simulink model "main_simulation"  (R2019b)
settings: Solver=VariableStepAuto  StartTime=0.0  StopTime=10.0  RelTol=1e-3
libraries: simulink x1
settings Model: Creator=LBRY-SVC-Patron  LastModifiedBy=logan
settings DataIOCC: ReturnWorkspaceOutputs=off
settings OptimizationCC: UseDivisionForNetSlopeComputation=on
settings DebuggingCC: ArithmeticOperatorsInVariantConditions=warning
settings SFSimCC: SimUseLocalCustomCode=off  CustomCodeUndefinedFunction=UseInterfaceOnly
settings RTWCC: RTWUseLocalCustomCode=off

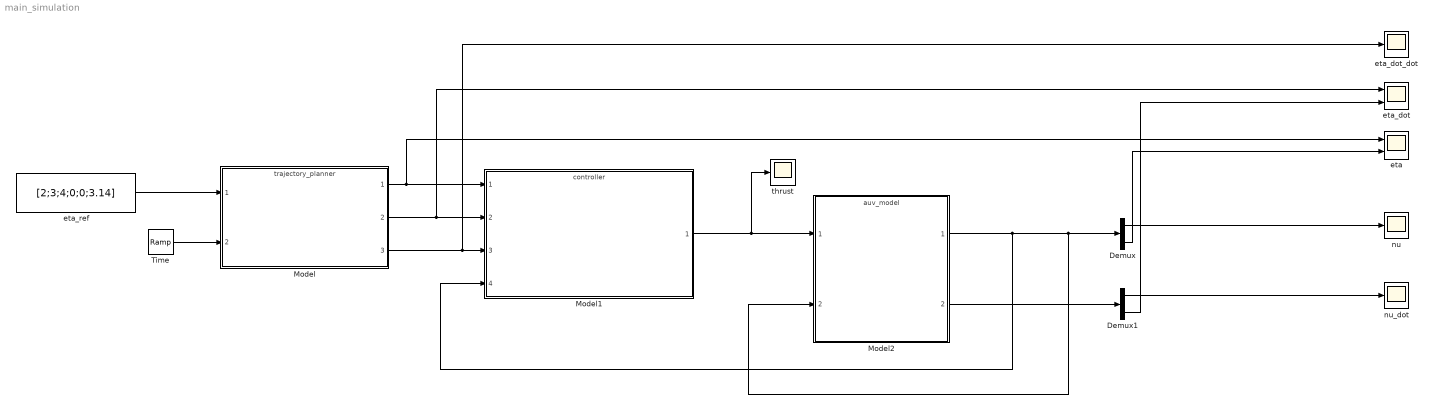
== system main_simulation ==
  Demux : Demux  Outputs=[6,6]
  Demux1 : Demux  Outputs=[6,6]
  Model : ModelReference  ModelNameDialog=trajectory_planner.slx  SimulationMode=Normal  ModelReferenceVersion=1.54
  Model1 : ModelReference  ModelNameDialog=controller.slx  SimulationMode=Normal  ModelReferenceVersion=1.79
  Model2 : ModelReference  ModelNameDialog=auv_model.slx  SimulationMode=Normal  ModelReferenceVersion=1.16
  "Time " : simulink/Sources/Ramp  slope=1  start=0  InitialOutput=0
  eta : Scope  NumInputPorts=2
  eta_dot : Scope  NumInputPorts=2
  eta_dot_dot : Scope
  eta_ref : Constant  Value=[2;3;4;0;0;3.14]
  nu : Scope
  nu_dot : Scope
  "thrust " : Scope
  wires:
  Model/1 -> Model1/1, eta/1
  Model/2 -> Model1/2, eta_dot/1
  "Time "/1 -> Model/2
  eta_ref/1 -> Model/1
  Model2/1 -> Model1/4, Demux/1, Model2/2
  Model1/1 -> "thrust "/1, Model2/1
  Model/3 -> Model1/3, eta_dot_dot/1
  Demux/1 -> nu/1
  Demux/2 -> eta/2
  Model2/2 -> Demux1/1
  Demux1/1 -> nu_dot/1
  Demux1/2 -> eta_dot/2
